simulink model "qss_example_optigear"  (Simulink 6.6)
settings: Solver=VariableStepDiscrete  StartTime=0.0  StopTime=1220  RelTol=1e-3
libraries: qss_tb_library x5
settings Model: Creator=csu  LastModifiedBy=csu  ExtModeAutoUpdateStatusClock=off
settings OptimizationCC: InlineInvariantSignals=on
settings DebuggingCC: SignalResolutionControl=TryResolveAllWithWarning  MultiTaskDSMMsg=warning  MultiTaskCondExecSysMsg=none  StrictBusMsg=None
settings RTWCC: IncludeERTFirstTime=on

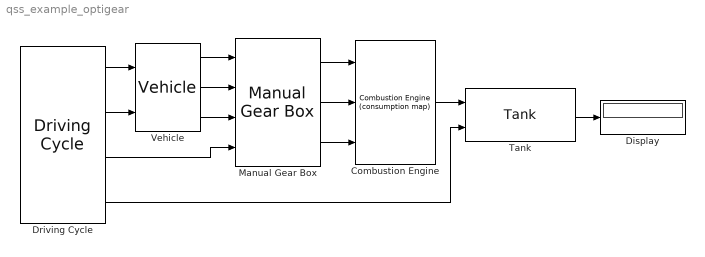
== system qss_example_optigear ==
  Combustion Engine : qss_tb_library/Energy Converter/Combustion Engine (consumption map)  Tag=combustion engine  SystemSampleTime=-1  engine_type=Otto  V_d=0.708  scale_CE=1  theta_CE=0.05  w_CE_idle=105  P_CE_idle=2600  P_aux=300  ENABLE_FUEL_CUTOFF=on  T_CE_cutoff=-5  P_CE_cutoff=0
  Display : Display
  Driving Cycle : qss_tb_library/Driving Cycle/Driving Cycle  Tag=cycle  SystemSampleTime=-1  cyclenr=Europe: NEDC  stepsize=1  autostop=on
  Manual Gear Box : qss_tb_library/Gear System/Manual Gear Box  Tag=transmission  SystemSampleTime=-1  i_1=first_gear  i_2=second_gear  i_3=third_gear  i_4=fourth_gear  i_5=fifth_gear  i_diff=1  e_GT=0.98  P_GT0=300  w_wheel_min=1
  Tank : qss_tb_library/Energy Source/Tank  Tag=tank  SystemSampleTime=-1  fuel=Gasoline  flag_cold_start=on
  Vehicle : qss_tb_library/Vehicle/Vehicle  Tag=vehicle  SystemSampleTime=-1  m_f=750  mt2m_f=5  A_f=1.8  d_wheel=0.5  cw=0.22  mu=0.008
  wires:
  Driving Cycle/1 -> Vehicle/1
  Vehicle/1 -> Manual Gear Box/1
  Vehicle/2 -> Manual Gear Box/2
  Vehicle/3 -> Manual Gear Box/3
  Driving Cycle/2 -> Vehicle/2
  Manual Gear Box/1 -> Combustion Engine/1
  Manual Gear Box/2 -> Combustion Engine/2
  Manual Gear Box/3 -> Combustion Engine/3
  Combustion Engine/1 -> Tank/1
  Driving Cycle/3 -> Manual Gear Box/4
  Driving Cycle/4 -> Tank/2
  Tank/1 -> Display/1
